simulink model "final"  (R2018b)
settings: Solver=ode3  StartTime=0.0  StopTime=10  RelTol=1e-3  EnableMultiTasking=on
libraries: legoev3lib x11
settings Model: FPTRunName=Active  ExtModeTrigDuration=2  Creator=jloehnertz  LastModifiedBy=jloehnertz
settings SolverCC: PositivePriorityOrder=on
settings DataIOCC: LimitDataPoints=on  SaveFormat=Array
settings OptimizationCC: ExpressionDepthLimit=2147483647  LifeSpan=Inf  MaxStackSize=64
settings DebuggingCC: UnderspecifiedInitializationDetection=Classic  MergeDetectMultiDrivingBlocksExec=none  FcnCallInpInsideContextMsg=warning  AllowSymbolicDim=off  StateNameClashWarn=warning  SFUnexpectedBacktrackingDiag=warning  SFNoUnconditionalDefaultTransitionDiag=warning  SFExecutionAtInitializationDiag=none
settings HardwareCC: ProdBitPerPointer=32  ProdBitPerSizeT=32  ProdBitPerPtrDiffT=32  ProdLargestAtomicInteger=Long  ProdWordSize=32  ProdHWDeviceType=ARM Compatible->ARM 9  UseEmbeddedCoderFeatures=off
settings ModelReferenceCC: PropagateSignalLabelsOutOfModel=off
settings SFSimCC: SimUseLocalCustomCode=off
settings RTWCC: SystemTargetFile=ert.tlc  HardwareBoard=LEGO MINDSTORMS EV3  TemplateMakefile=ert_default_tmf  GenerateReport=on  RTWVerbose=off  RTWUseLocalCustomCode=off  Toolchain=Sourcery G++ Lite v2009q3  BuildConfiguration=Faster Runs  LaunchReport=on
settings CodeAppCC: ForceParamTrailComments=on  OperatorAnnotations=on  StateflowObjectComments=on  MATLABSourceComments=on
settings ERTTargetCC: MultiwordLength=2048  ERTCustomFileBanners=off  SupportContinuousTime=on  SupportNonInlinedSFcns=on  RemoveResetFunc=off  SupportVariableSizeSignals=on  ModelStepFunctionPrototypeControlCompliant=off
settings ConfigComp: CovMetricSettings=dw  CovHtmlReporting=on  CovSaveCumulativeToWorkspaceVar=on  CovSaveSingleToWorkspaceVar=on  CovExternalEMLEnable=off  CovSFcnEnable=off

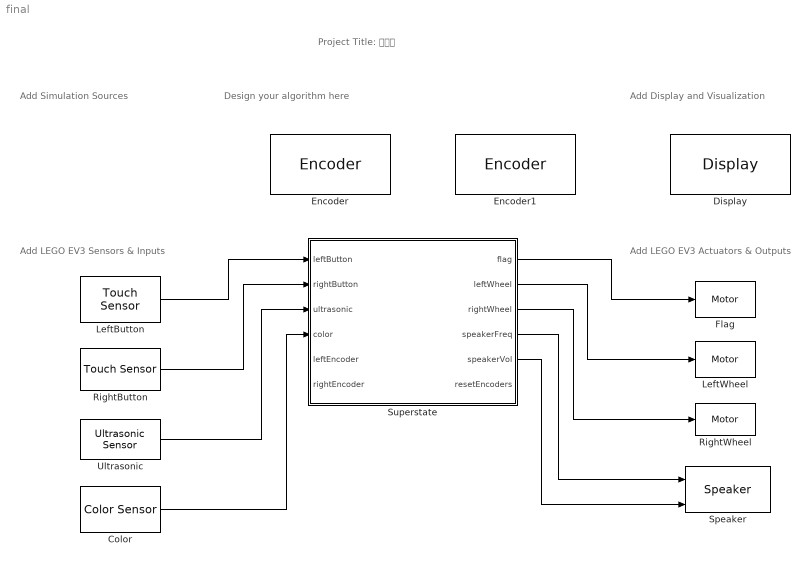
== system final ==
  note: Project Title: 🔮🐙🏝️
  note: Add LEGO EV3 Sensors & Inputs
  note: Add LEGO EV3 Actuators & Outputs
  note: Add Display and Visualization
  note: Design your algorithm here
  note: Add Simulation Sources
  Color : legoev3lib/Color Sensor  portNumber=1  mode=Color  sampleTime=0.1
      settings: SourceProductName=Simulink Support Package for LEGO MINDSTORMS EV3 Hardware  SourceProductBaseCode=LEGOEV3
  Display : legoev3lib/Display  slcdLine=1  slcdFormat=Decimal
      settings: SourceProductName=Simulink Support Package for LEGO MINDSTORMS EV3 Hardware  SourceProductBaseCode=LEGOEV3
  Encoder : legoev3lib/Encoder  portNumber=A  opMode=Reset by external signal  sampleTime=0.1
      settings: SourceProductName=Simulink Support Package for LEGO MINDSTORMS EV3 Hardware  SourceProductBaseCode=LEGOEV3
  Encoder1 : legoev3lib/Encoder  portNumber=A  opMode=Reset by external signal  sampleTime=0.1
      settings: SourceProductName=Simulink Support Package for LEGO MINDSTORMS EV3 Hardware  SourceProductBaseCode=LEGOEV3
  Flag : legoev3lib/Motor  sportNumber=B  sstopAction=Brake
  LeftButton : legoev3lib/Touch Sensor  portNumber=1  sampleTime=0.1
      settings: SourceProductName=Simulink Support Package for LEGO MINDSTORMS EV3 Hardware  SourceProductBaseCode=LEGOEV3
  LeftWheel : legoev3lib/Motor  sportNumber=A  sstopAction=Brake
  RightButton : legoev3lib/Touch Sensor  portNumber=2  sampleTime=0.1
      settings: SourceProductName=Simulink Support Package for LEGO MINDSTORMS EV3 Hardware  SourceProductBaseCode=LEGOEV3
  RightWheel : legoev3lib/Motor  sportNumber=C  sstopAction=Brake
  Speaker : legoev3lib/Speaker  sinputMode=Frequency and volume  sspeakerFreq=100  sspeakerVolume=50  sspeakerDuration=100
      settings: SourceProductName=Simulink Support Package for LEGO MINDSTORMS EV3 Hardware  SourceProductBaseCode=LEGOEV3
  Superstate : Stateflow chart  TreatAsAtomicUnit=on
  Ultrasonic : legoev3lib/Ultrasonic Sensor  PortNumber=1  sampleTime=0.1
      settings: SourceProductName=Simulink Support Package for LEGO MINDSTORMS EV3 Hardware  SourceProductBaseCode=LEGOEV3
  wires:
  LeftButton/1 -> Superstate/1(leftButton)
  RightButton/1 -> Superstate/2(rightButton)
  Superstate/1(flag) -> Flag/1
  Superstate/3(rightWheel) -> RightWheel/1
  Superstate/2(leftWheel) -> LeftWheel/1
  Superstate/4(speakerFreq) -> Speaker/1
  Superstate/5(speakerVol) -> Speaker/2
  Ultrasonic/1 -> Superstate/3(ultrasonic)
  Color/1 -> Superstate/4(color)

== stateflow chart final/Superstate ==
  state Manual
    state RESET
    state TURNLEFT
      entry:
      leftWheel = 23
      rightWheel = -23
    state MANUAL
      entry:
      leftWheel = 0;
      rightWheel = 0;
    state AUTONOMOUS
      entry:
      send(autonomous)
    state HOLD
    state STOP
    state FORWARD
      entry:
      leftWheel = 30;
      rightWheel = 30;
    state TURNRIGHT
      entry:
      leftWheel = -23
      rightWheel = 23
    RESET -> MANUAL [order 1] : after(1, sec)
    RESET -> AUTONOMOUS [order 2] : [not(leftButton == 1 & rightButton == 1)]
    TURNLEFT -> MANUAL : [not(leftButton == 1 & rightButton == 0)]
    MANUAL -> TURNLEFT [order 1] : [leftButton == 1 & rightButton == 0]
    (default) -> MANUAL
    MANUAL -> HOLD [order 3] : [leftButton == 1 & rightButton == 1]
    HOLD -> AUTONOMOUS [order 2] : after(1, sec)
    HOLD -> FORWARD [order 1] : [not(leftButton == 1 & rightButton == 1)]
    STOP -> MANUAL : [leftButton == 0 & rightButton == 0]
    FORWARD -> STOP : [not(leftButton == 0 & rightButton == 0)]
    TURNRIGHT -> MANUAL : [not(leftButton == 0 & rightButton == 1)]
    MANUAL -> TURNRIGHT [order 2] : [leftButton == 0 & rightButton == 1]
  state Autonomous
    state Approach
      state Start
        entry:
        leftWheel = 20;
        rightWheel = 20;
      state Wait
        entry:
        leftWheel = 0;
        rightWheel = 0;
      state Exit
        entry:
        send(exitApproach)
      (default) -> Start
      Start -> Wait : [ultrasonic < stopDistance]
      Wait -> Exit : after(5, sec)
    state flee1
      state BeepAndTurn
        entry:
        speakerFreq = 600;
        speakerVol = 100;
        leftWheel = 100;
        rightWheel = -100;
      state ResetEncoders
        entry:
        resetEncoders = 1;
        exit:
        resetEncoders = 0;
      state PauseRealQuick
        entry:
        leftWheel = 0;
        rightWheel = 0;
      state MoveForward
        entry:
        speakerFreq = 0;
        speakerVol = 0;
        leftWheel = 100;
        rightWheel = 100;
      state BeepStop
        entry:
        speakerFreq = 0;
        speakerVol = 0;
      state Beep
        entry:
        speakerFreq = 600;
        speakerVol = 100;
      state StopRobot
        entry:
        leftWheel = 0;
        rightWheel = 0;
      (default) -> BeepAndTurn
      BeepAndTurn -> PauseRealQuick : [leftEncoder - rightEncoder > 3 * 90]
      ResetEncoders -> BeepAndTurn
      PauseRealQuick -> MoveForward : after(0.2, sec)
      MoveForward -> StopRobot : after(0.5, sec)
      StopRobot -> Beep : after(0.5, sec)
      Beep -> BeepStop : after(0.5, sec)
    (default) -> Approach
    Approach -> (junction 21) : [exitApproach]
  (default) -> Manual
  Autonomous -> RESET : [leftButton == 1 & rightButton == 1]
  Manual -> (history) : [autonomous]
  data: leftButton input; rightButton input; flag output; leftWheel output; rightWheel output; speakerFreq output; speakerVol output; ultrasonic input; color input; stopDistance constant double =20; resetEncoders output; leftEncoder input; rightEncoder input
  events: exitApproach local FUNCTION_CALL_EVENT; autonomous local FUNCTION_CALL_EVENT
